simulink model "zad5"  (R2022b)
settings: Solver=VariableStepAuto  StartTime=0.0  StopTime=200  RelTol=1e-3
values from neighbouring files (symbols this model uses):
  a0 = 0.000641026    [parameters.m]
  a1 = 0.0224359    [parameters.m]
  a2 = 0.260256    [parameters.m]
  Tp = 1    [parameters.m]
settings Model: Creator=Mat  LastModifiedBy=Mat

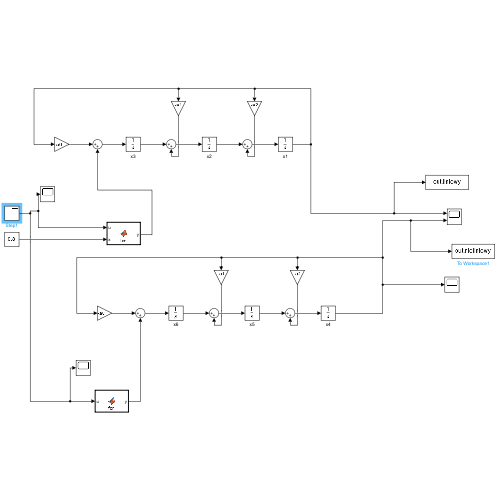
[thumbnail: Simulink's stored preview of the top-level diagram]
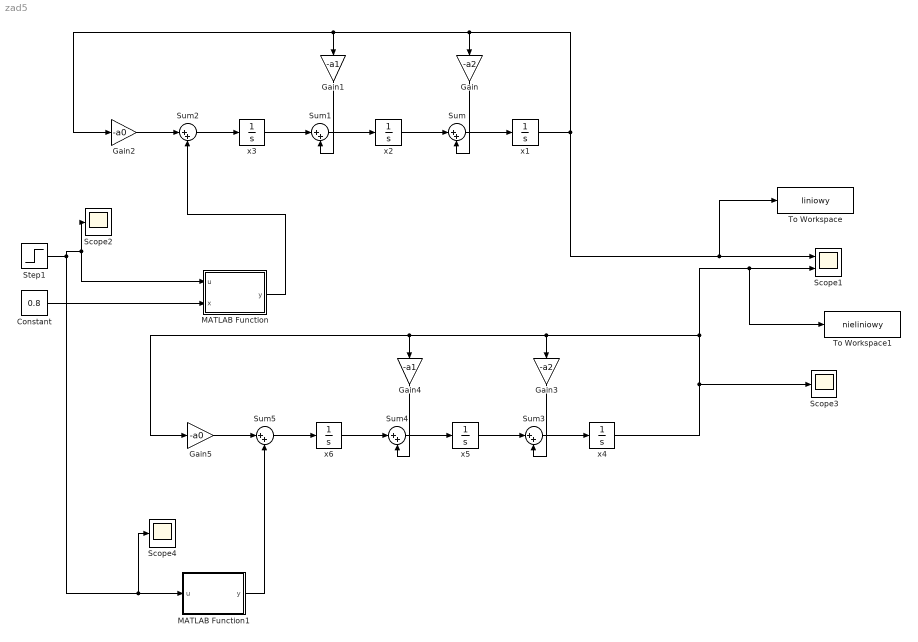
== system zad5 ==
  Constant : Constant  Value=0.8
  Gain : Gain  Gain=-a2
  Gain1 : Gain  Gain=-a1
  Gain2 : Gain  Gain=-a0
  Gain3 : Gain  Gain=-a2
  Gain4 : Gain  Gain=-a1
  Gain5 : Gain  Gain=-a0
  MATLAB Function : MATLAB Function  TreatAsAtomicUnit=on
  MATLAB Function1 : MATLAB Function  TreatAsAtomicUnit=on
  Scope1 : Scope  NumInputPorts=2
  Scope2 : Scope
  Scope3 : Scope
  Scope4 : Scope
  Step1 : Step  Time=30  Before=-1  After=0.9  SampleTime=Tp
  Sum{,1..5} (6 alike) : Sum  Inputs=|++
  To Workspace : ToWorkspace  VariableName=liniowy  SaveFormat=Timeseries  SampleTime=-1
  To Workspace1 : ToWorkspace  VariableName=nieliniowy  SaveFormat=Timeseries  SampleTime=-1
  x{1..6} (6 alike) : Integrator
  wires:
  x3/1 -> Sum1/1
  Gain2/1 -> Sum2/1
  Gain1/1 -> Sum1/2
  Gain/1 -> Sum/2
  Sum/1 -> x1/1
  Sum2/1 -> x3/1
  Sum1/1 -> x2/1
  x2/1 -> Sum/1
  x1/1 -> To Workspace/1, Scope1/1, Gain1/1, Gain2/1, Gain/1
  Constant/1 -> MATLAB Function/2(x)
  MATLAB Function/1(y) -> Sum2/2
  MATLAB Function1/1(y) -> Sum5/2
  Sum4/1 -> x5/1
  Gain5/1 -> Sum5/1
  x6/1 -> Sum4/1
  Gain4/1 -> Sum4/2
  Step1/1 -> MATLAB Function/1(u), Scope2/1, Scope4/1, MATLAB Function1/1(u)
  x5/1 -> Sum3/1
  Sum3/1 -> x4/1
  Sum5/1 -> x6/1
  Gain3/1 -> Sum3/2
  x4/1 -> Scope3/1, To Workspace1/1, Scope1/2, Gain4/1, Gain5/1, Gain3/1

== matlab function zad5/MATLAB Function ==
  data: u input; y output; x input
function y  = fcn(u, x)
b0 = 0.000897436;
alfa1 = 1.3;
alfa2 = 1.1;
alfa3 = -1.15;
alfa4 = -0.9;

y = b0*((alfa1*x+alfa2*x^2+alfa3*x^3+alfa4*x^4) + ...
    (alfa1*2*alfa2*x + 3*alfa3*x^2 + 4*alfa4*x^3) * (u - x));
end

== matlab function zad5/MATLAB Function1 ==
  data: u input; y output
function y = fcn(u)
b0 = 0.000897436;
alfa1 = 1.3;
alfa2 = 1.1;
alfa3 = -1.15;
alfa4 = -0.9;
y = b0*(alfa1*u+alfa2*u^2+alfa3*u^3+alfa4*u^4);
end
